simulink model "sistema"  (R2024b)
settings: Solver=VariableStepAuto  StartTime=0.0  StopTime=10.0  RelTol=1e-3
settings Model: Creator=brandon  LastModifiedBy=brandon

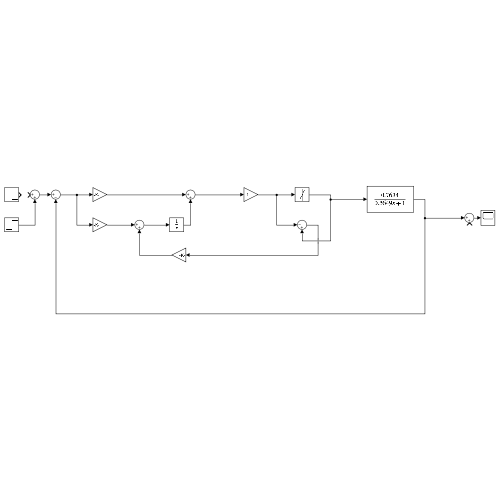
[thumbnail: Simulink's stored preview of the top-level diagram]
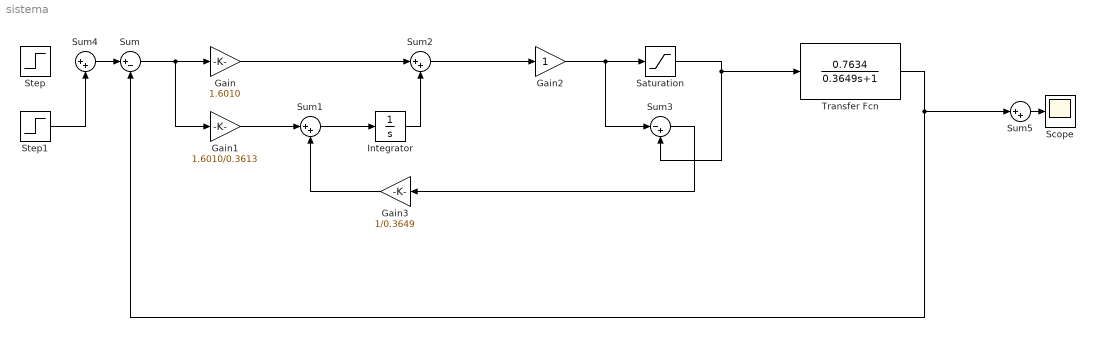
== system sistema ==
  Gain : Gain  Gain=1.6010
  Gain1 : Gain  Gain=1.6010/0.3613
  Gain2 : Gain
  Gain3 : Gain  Gain=1/0.3649
  Integrator : Integrator
  Saturation : Saturate  UpperLimit=500  LowerLimit=-500
  Scope : Scope
  Step : Step  Time=2  Before=150  After=120  SampleTime=0.01
  Step1 : Step  Time=7  Before=120  After=150  SampleTime=0.01
  Sum : Sum  Inputs=|+-
  Sum{1..2,4..5} (4 alike) : Sum  Inputs=|++
  Sum3 : Sum  Inputs=|-+
  Transfer Fcn : TransferFcn  Numerator=[0.7634]  Denominator=[0.3649 1]
  wires:
  Gain2/1 -> Sum3/1, Saturation/1
  Saturation/1 -> Sum3/2, Transfer Fcn/1
  Sum3/1 -> Gain3/1
  Gain3/1 -> Sum1/2
  Gain1/1 -> Sum1/1
  Sum1/1 -> Integrator/1
  Integrator/1 -> Sum2/2
  Sum2/1 -> Gain2/1
  Gain/1 -> Sum2/1
  Transfer Fcn/1 -> Sum5/1, Sum/2
  Sum/1 -> Gain1/1, Gain/1
  Sum4/1 -> Sum/1
  Sum5/1 -> Scope/1
  Step1/1 -> Sum4/2
